simulink model "w1que1"  (R2020b)
settings: Solver=VariableStepAuto  StartTime=0.0  StopTime=10.0  RelTol=1e-3
settings Model: Creator=ANUJA  LastModifiedBy=ANUJA

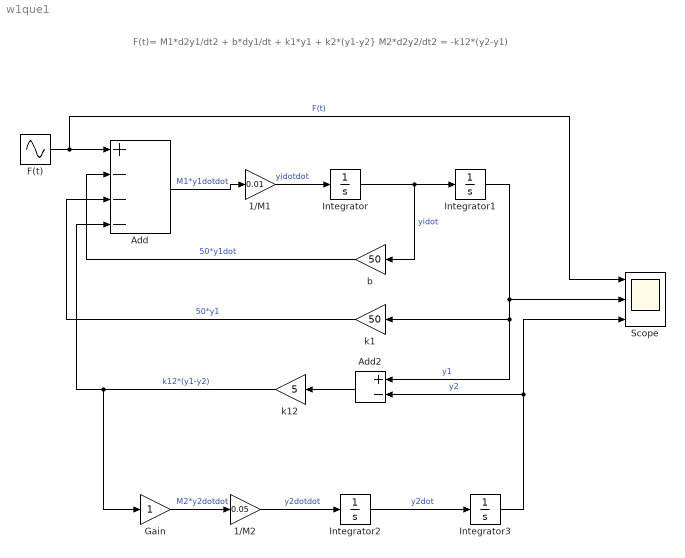
== system w1que1 ==
  note: F(t)= M1*d2y1/dt2 + b*dy1/dt + k1*y1 + k2*(y1-y2}
      |
      | M2*d2y2/dt2 = -k12*(y2-y1)
  1/M1 : Gain  Gain=0.01
  1/M2 : Gain  Gain=0.05
  Add : Sum  Inputs=+---
  Add2 : Sum  Inputs=+-
  F(t) : Sin  Amplitude=2  Frequency=10  SampleTime=0
  Gain : Gain
  Integrator{,1..3} (4 alike) : Integrator
  Scope : Scope  NumInputPorts=3
  b : Gain  Gain=50
  k1 : Gain  Gain=50
  k12 : Gain  Gain=5
  wires:
  b/1 -> Add/2  "50*y1dot"
  Gain/1 -> 1/M2/1  "M2*y2dotdot"
  Add/1 -> 1/M1/1  "M1*y1dotdot"
  k12/1 -> Gain/1, Add/4  "k12*(y1-y2)"
  Integrator3/1 -> Scope/3, Add2/2  "y2"
  Add2/1 -> k12/1
  k1/1 -> Add/3  "50*y1"
  Integrator1/1 -> Add2/1, k1/1, Scope/2  "y1"
  Integrator/1 -> b/1, Integrator1/1  "yidot"
  1/M2/1 -> Integrator2/1  "y2dotdot"
  F(t)/1 -> Scope/1, Add/1  "F(t)"
  1/M1/1 -> Integrator/1  "yidotdot"
  Integrator2/1 -> Integrator3/1  "y2dot"
